simulink model "stochasticJumplinearSystem_simple_test_simulink"  (R2015a)
settings: Solver=ode3  StartTime=0.0  StopTime=1000.0  FixedStep=1e-3  RelTol=1e-3
undefined symbols (not defined in the file or in its folder): pow
libraries: simulink x1
settings Model: Creator=ak22emur  LastModifiedBy=ak22emur

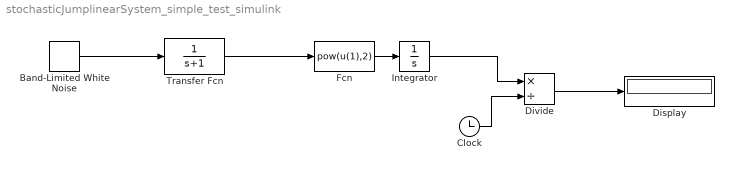
== system stochasticJumplinearSystem_simple_test_simulink ==
  Band-Limited White Noise : simulink/Sources/Band-Limited White Noise  Cov=1  Ts=1e-3  seed=[23341]
  Clock : Clock
  Display : Display
  Divide : Product  Inputs=*/
  Fcn : Fcn  Expr=pow(u(1),2)
  Integrator : Integrator
  Transfer Fcn : TransferFcn  Denominator=[1 1]
  wires:
  Band-Limited White Noise/1 -> Transfer Fcn/1
  Transfer Fcn/1 -> Fcn/1
  Fcn/1 -> Integrator/1
  Integrator/1 -> Divide/1
  Clock/1 -> Divide/2
  Divide/1 -> Display/1
